simulink model "Test"  (Simulink 7.9)
settings: Solver=ode4  StartTime=0.0  StopTime=3.3  FixedStep=1e-5  MaxStep=1e-4  RelTol=1e-5
libraries: simulink x2
settings Model: Creator=oli  LastModifiedBy=oli
settings DataIOCC: SaveFormat=StructureWithTime  SaveState=on

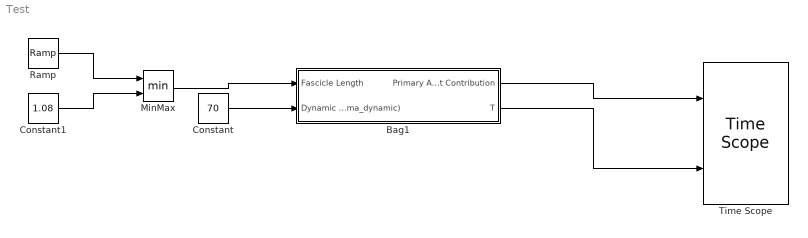
== system Test ==
  Bag1 : Subsystem
  Constant : Constant  Value=70
  Constant1 : Constant  Value=1.08
  MinMax : MinMax  Inputs=2
  Ramp : simulink/Sources/Ramp  slope=.11  start=1  X0=0.95
  Time Scope : TimeScope  NumInputPorts=2
      settings: CopyFcn=scopeextensions.ScopeBlock.callback(gcbh, 'onBlockCopy', gcbh);  DeleteFcn=scopeextensions.ScopeBlock.callback(gcbh, 'onBlockDelete');  PreSaveFcn=scopeextensions.ScopeBlock.callback(gcbh, 'onModelSave');  NameChangeFcn=scopeextensions.ScopeBlock.callback(gcbh, 'onBlockRename');  OpenFcn=scopeextensions.SrcWiredSL.coreBlockCommand('Open',gcbh)  CloseFcn=scopeextensions.ScopeBlock.callback(gcbh, 'onBlockClose');  PreDeleteFcn=scopeextensions.ScopeBlock.callback(gcbh, 'onBlockPreDelete');
  wires:
  Constant/1 -> Bag1/2(Dynamic Fusimotor (Gamma_dynamic))
  Ramp/1 -> MinMax/1
  Constant1/1 -> MinMax/2
  Bag1/2(T) -> Time Scope/2
  Bag1/1(Primary Afferent Contribution) -> Time Scope/1
  MinMax/1 -> Bag1/1(Fascicle Length)

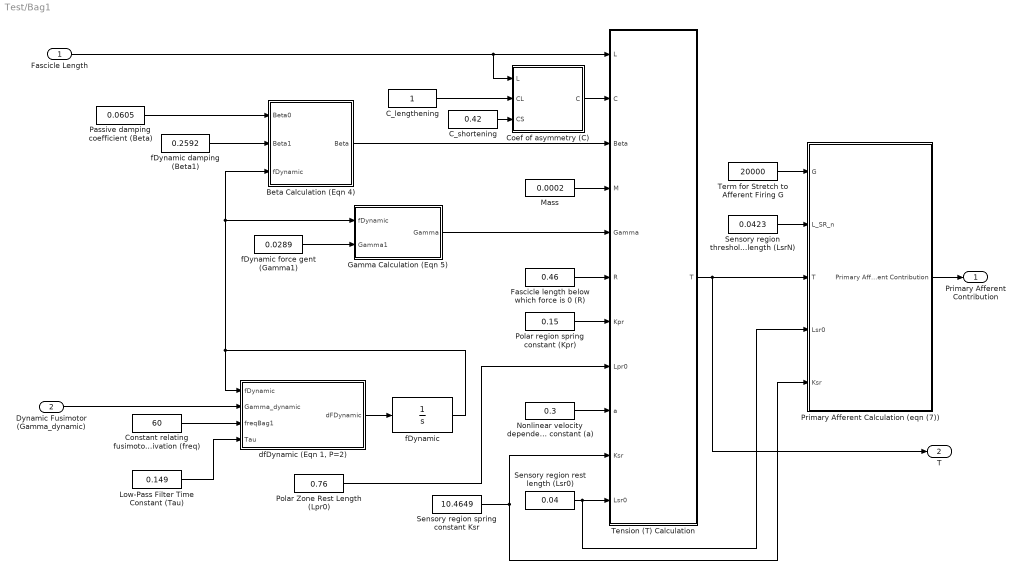
== system Test/Bag1 ==
  Fascicle Length : Inport
  Dynamic Fusimotor (Gamma_dynamic) : Inport  Port=2
  Beta Calculation (Eqn 4) : Subsystem
  C_lengthening : Constant
  C_shortening : Constant  Value=0.42
  Coef of asymmetry (C) : Subsystem
  Constant relating fusimotor frequency to activation (freq) : Constant  Value=60
  Fascicle length below which force is 0 (R) : Constant  Value=0.46
  Gamma Calculation (Eqn 5) : Subsystem
  Low-Pass Filter Time Constant (Tau) : Constant  Value=0.149
  Mass : Constant  Value=0.0002
  Nonlinear velocity dependence power constant (a) : Constant  Value=0.3
  Passive damping coefficient (Beta) : Constant  Value=0.0605
  Polar Zone Rest Length (Lpr0) : Constant  Value=0.76
  Polar region spring constant (Kpr) : Constant  Value=0.15
  Primary Afferent Calculation (eqn (7)) : Subsystem
  Sensory region rest length (Lsr0) : Constant  Value=0.04
  Sensory region spring constant Ksr : Constant  Value=10.4649
  Sensory region threshold length (LsrN) : Constant  Value=0.0423
  "Tension (T) Calculation " : Subsystem
  Term for Stretch to Afferent Firing G : Constant  Value=20000
  "dfDynamic (Eqn 1, P=2)" : Subsystem
  fDynamic : Integrator
  fDynamic damping (Beta1) : Constant  Value=0.2592
  fDynamic force gent (Gamma1) : Constant  Value=0.0289
  Primary Afferent Contribution : Outport
  T : Outport  Port=2
  wires:
  Polar Zone Rest Length (Lpr0)/1 -> "Tension (T) Calculation "/8(Lpr0)
  fDynamic/1 -> Beta Calculation (Eqn 4)/3(fDynamic), Gamma Calculation (Eqn 5)/1(fDynamic), "dfDynamic (Eqn 1, P=2)"/1(fDynamic)
  "dfDynamic (Eqn 1, P=2)"/1(dFDynamic) -> fDynamic/1
  Dynamic Fusimotor (Gamma_dynamic)/1 -> "dfDynamic (Eqn 1, P=2)"/2(Gamma_dynamic)
  Low-Pass Filter Time Constant (Tau)/1 -> "dfDynamic (Eqn 1, P=2)"/4(Tau)
  Constant relating fusimotor frequency to activation (freq)/1 -> "dfDynamic (Eqn 1, P=2)"/3(freqBag1)
  Primary Afferent Calculation (eqn (7))/1(Primary Afferent Contribution) -> Primary Afferent Contribution/1
  "Tension (T) Calculation "/1(T) -> Primary Afferent Calculation (eqn (7))/3(T), T/1
  Term for Stretch to Afferent Firing G/1 -> Primary Afferent Calculation (eqn (7))/1(G)
  Sensory region spring constant Ksr/1 -> Primary Afferent Calculation (eqn (7))/5(Ksr), "Tension (T) Calculation "/10(Ksr)
  Sensory region rest length (Lsr0)/1 -> Primary Afferent Calculation (eqn (7))/4(Lsr0), "Tension (T) Calculation "/11(Lsr0)
  Sensory region threshold length (LsrN)/1 -> Primary Afferent Calculation (eqn (7))/2(L_SR_n)
  Passive damping coefficient (Beta)/1 -> Beta Calculation (Eqn 4)/1(Beta0)
  Beta Calculation (Eqn 4)/1(Beta) -> "Tension (T) Calculation "/3(Beta)
  fDynamic damping (Beta1)/1 -> Beta Calculation (Eqn 4)/2(Beta1)
  Mass/1 -> "Tension (T) Calculation "/4(M)
  fDynamic force gent (Gamma1)/1 -> Gamma Calculation (Eqn 5)/2(Gamma1)
  Fascicle Length/1 -> "Tension (T) Calculation "/1(L), Coef of asymmetry (C)/1(L)
  Fascicle length below which force is 0 (R)/1 -> "Tension (T) Calculation "/6(R)
  Gamma Calculation (Eqn 5)/1(Gamma) -> "Tension (T) Calculation "/5(Gamma)
  C_lengthening/1 -> Coef of asymmetry (C)/2(CL)
  C_shortening/1 -> Coef of asymmetry (C)/3(CS)
  Coef of asymmetry (C)/1(C) -> "Tension (T) Calculation "/2(C)
  Nonlinear velocity dependence power constant (a)/1 -> "Tension (T) Calculation "/9(a)
  Polar region spring constant (Kpr)/1 -> "Tension (T) Calculation "/7(Kpr)

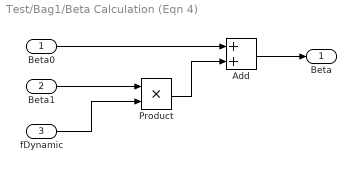
== system Test/Bag1/Beta Calculation (Eqn 4) ==
  Beta0 : Inport
  Beta1 : Inport  Port=2
  fDynamic : Inport  Port=3
  Add : Sum
  Product : Product  RndMeth=Zero
  Beta : Outport
  wires:
  Beta1/1 -> Product/1
  fDynamic/1 -> Product/2
  Add/1 -> Beta/1
  Beta0/1 -> Add/1
  Product/1 -> Add/2

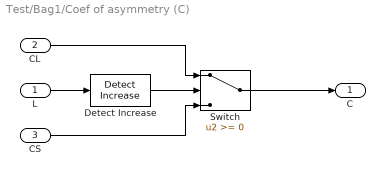
== system Test/Bag1/Coef of asymmetry (C) ==
  L : Inport
  CL : Inport  Port=2
  CS : Inport  Port=3
  Detect Increase : simulink/Logic and Bit Operations/Detect Increase  vinit=0.0  InputProcessing=Inherited  OutDataTypeStr=uint8
  Switch : Switch
  C : Outport
  wires:
  CL/1 -> Switch/1
  CS/1 -> Switch/3
  Switch/1 -> C/1
  L/1 -> Detect Increase/1
  Detect Increase/1 -> Switch/2

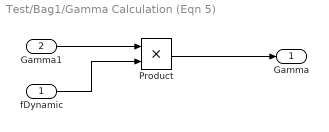
== system Test/Bag1/Gamma Calculation (Eqn 5) ==
  fDynamic : Inport
  Gamma1 : Inport  Port=2
  Product : Product  RndMeth=Zero
  Gamma : Outport
  wires:
  Product/1 -> Gamma/1
  Gamma1/1 -> Product/1
  fDynamic/1 -> Product/2

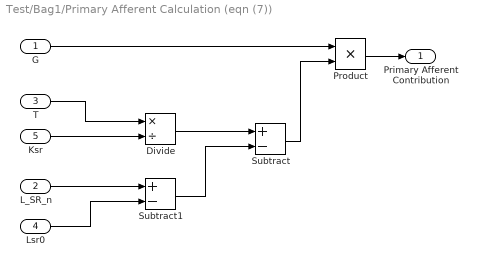
== system Test/Bag1/Primary Afferent Calculation (eqn (7)) ==
  G : Inport
  L_SR_n : Inport  Port=2
  T : Inport  Port=3
  Lsr0 : Inport  Port=4
  Ksr : Inport  Port=5
  Divide : Product  Inputs=*/
  Product : Product  RndMeth=Zero
  Subtract : Sum  Inputs=+-
  Subtract1 : Sum  Inputs=+-
  Primary Afferent Contribution : Outport
  wires:
  G/1 -> Product/1
  Product/1 -> Primary Afferent Contribution/1
  Subtract/1 -> Product/2
  T/1 -> Divide/1
  Ksr/1 -> Divide/2
  Divide/1 -> Subtract/1
  L_SR_n/1 -> Subtract1/1
  Lsr0/1 -> Subtract1/2
  Subtract1/1 -> Subtract/2

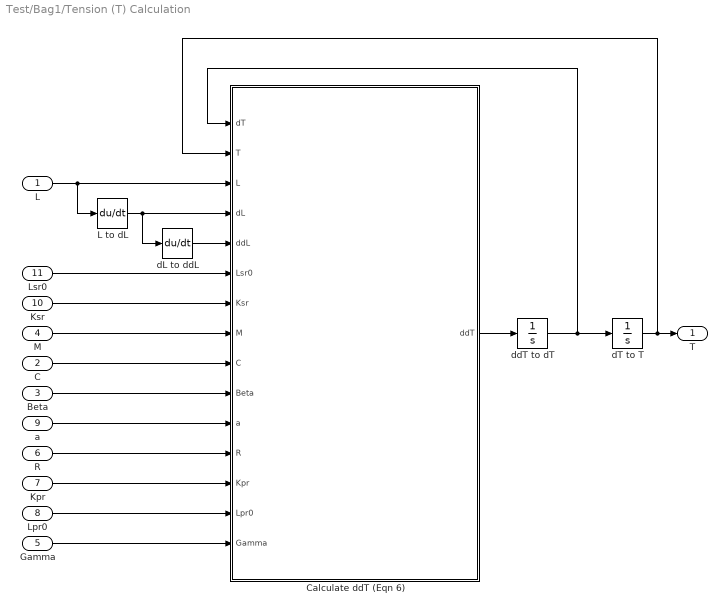
== system Test/Bag1/Tension (T) Calculation  ==
  L : Inport
  C : Inport  Port=2
  Beta : Inport  Port=3
  M : Inport  Port=4
  Gamma : Inport  Port=5
  R : Inport  Port=6
  Kpr : Inport  Port=7
  Lpr0 : Inport  Port=8
  a : Inport  Port=9
  Ksr : Inport  Port=10
  Lsr0 : Inport  Port=11
  Calculate ddT (Eqn 6) : MATLAB Function  TreatAsAtomicUnit=on
  L to dL : Derivative  CoefficientInTFapproximation=Inf
  dL to ddL : Derivative  CoefficientInTFapproximation=Inf
  dT to T : Integrator
  ddT to dT : Integrator
  T : Outport
  wires:
  L/1 -> Calculate ddT (Eqn 6)/3(L), L to dL/1
  Lsr0/1 -> Calculate ddT (Eqn 6)/6(Lsr0)
  Gamma/1 -> Calculate ddT (Eqn 6)/15(Gamma)
  Kpr/1 -> Calculate ddT (Eqn 6)/13(Kpr)
  a/1 -> Calculate ddT (Eqn 6)/11(a)
  C/1 -> Calculate ddT (Eqn 6)/9(C)
  Lpr0/1 -> Calculate ddT (Eqn 6)/14(Lpr0)
  Beta/1 -> Calculate ddT (Eqn 6)/10(Beta)
  Ksr/1 -> Calculate ddT (Eqn 6)/7(Ksr)
  M/1 -> Calculate ddT (Eqn 6)/8(M)
  R/1 -> Calculate ddT (Eqn 6)/12(R)
  Calculate ddT (Eqn 6)/1(ddT) -> ddT to dT/1
  ddT to dT/1 -> dT to T/1, Calculate ddT (Eqn 6)/1(dT)
  dT to T/1 -> T/1, Calculate ddT (Eqn 6)/2(T)
  L to dL/1 -> Calculate ddT (Eqn 6)/4(dL), dL to ddL/1
  dL to ddL/1 -> Calculate ddT (Eqn 6)/5(ddL)

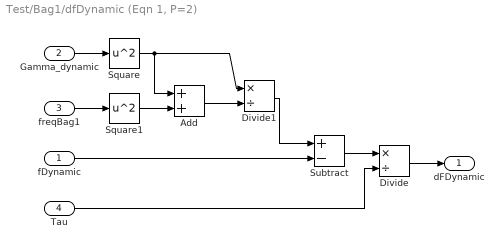
== system Test/Bag1/dfDynamic (Eqn 1, P=2) ==
  fDynamic : Inport
  Gamma_dynamic : Inport  Port=2
  freqBag1 : Inport  Port=3
  Tau : Inport  Port=4
  Add : Sum
  Divide : Product  Inputs=*/
  Divide1 : Product  Inputs=*/
  Square : Math  Operator=square  SaturateOnIntegerOverflow=on
  Square1 : Math  Operator=square  SaturateOnIntegerOverflow=on
  Subtract : Sum  Inputs=+-
  dFDynamic : Outport
  wires:
  Divide/1 -> dFDynamic/1
  Tau/1 -> Divide/2
  Subtract/1 -> Divide/1
  fDynamic/1 -> Subtract/2
  Divide1/1 -> Subtract/1
  Add/1 -> Divide1/2
  Gamma_dynamic/1 -> Square/1
  Square/1 -> Divide1/1, Add/1
  freqBag1/1 -> Square1/1
  Square1/1 -> Add/2

== matlab function Bag1/Tension (T) Calculation /Calculate ddT (Eqn 6) ==
  data: dT input double; T input double; L input double; dL input double; ddL input double; Lsr0 input double; Ksr input double; ddT output double; M input double; C input double; Beta input double; a input double; R input double; Kpr input double; Lpr0 input double; Gamma input double
function ddT = Calculate_ddT(dT, T, L, dL, ddL, Lsr0, Ksr, M, C, Beta, a, R, Kpr, Lpr0, Gamma)

    LTerm = L - Lsr0 - T/Ksr;

    ddT = Ksr/M * (...
            C * Beta * sign(dL - dT/Ksr) * abs(dL - dT/Ksr)^a * (LTerm - R) ...
            + Kpr * (LTerm - Lpr0) ...
            + M * ddL ...
            + Gamma ...
            - T);
end
